simulink model "InjCrv_MI11"  (R2016b)
settings: configuration reference "CodeGenConfigSet" (kept outside this file)
values from neighbouring files (symbols this model uses):
  InjCrv_phiMI1Bas1EOM0_MAP = Calibration.Parameter    [init_InjCrv_MI1.m]    (also in init_InjCrv_MI1_SIL.m = Simulink.Parameter)
  InjCrv_phiMI1Bas1EOM0_MAPX = Calibration.Parameter    [init_InjCrv_MI1.m]    (also in init_InjCrv_MI1_SIL.m = Simulink.Parameter)
  InjCrv_phiMI1Bas1EOM0_MAPY = Calibration.Parameter    [init_InjCrv_MI1.m]    (also in init_InjCrv_MI1_SIL.m = Simulink.Parameter)
  InjCrv_phiMI1Bas2EOM0_MAP = Calibration.Parameter    [init_InjCrv_MI1.m]    (also in init_InjCrv_MI1_SIL.m = Simulink.Parameter)
  InjCrv_phiMI1Bas2EOM0_MAPX = Calibration.Parameter    [init_InjCrv_MI1.m]    (also in init_InjCrv_MI1_SIL.m = Simulink.Parameter)
  InjCrv_phiMI1Bas2EOM0_MAPY = Calibration.Parameter    [init_InjCrv_MI1.m]    (also in init_InjCrv_MI1_SIL.m = Simulink.Parameter)
  InjCrv_phiMI1Max1EOM0_MAP = Calibration.Parameter    [init_InjCrv_MI1.m]    (also in init_InjCrv_MI1_SIL.m = Simulink.Parameter)
  InjCrv_phiMI1Max1EOM0_MAPX = Calibration.Parameter    [init_InjCrv_MI1.m]    (also in init_InjCrv_MI1_SIL.m = Simulink.Parameter)
  InjCrv_phiMI1Max1EOM0_MAPY = Calibration.Parameter    [init_InjCrv_MI1.m]    (also in init_InjCrv_MI1_SIL.m = Simulink.Parameter)
  InjCrv_phiMI1Max2EOM0_MAP = Calibration.Parameter    [init_InjCrv_MI1.m]    (also in init_InjCrv_MI1_SIL.m = Simulink.Parameter)
  InjCrv_phiMI1Max2EOM0_MAPX = Calibration.Parameter    [init_InjCrv_MI1.m]    (also in init_InjCrv_MI1_SIL.m = Simulink.Parameter)
  InjCrv_phiMI1Max2EOM0_MAPY = Calibration.Parameter    [init_InjCrv_MI1.m]    (also in init_InjCrv_MI1_SIL.m = Simulink.Parameter)
  InjCrv_phiMI1Min_C = Calibration.Parameter    [init_InjCrv_MI1.m]    (also in init_InjCrv_MI1_SIL.m = Simulink.Parameter)
  InjCrv_phiMI1StrtBase_MAP = Calibration.Parameter    [init_InjCrv_MI1.m]    (also in init_InjCrv_MI1_SIL.m = Simulink.Parameter)
  InjCrv_phiMI1StrtBase_MAPX = Calibration.Parameter    [init_InjCrv_MI1.m]    (also in init_InjCrv_MI1_SIL.m = Simulink.Parameter)
  InjCrv_phiMI1StrtBase_MAPY = Calibration.Parameter    [init_InjCrv_MI1.m]    (also in init_InjCrv_MI1_SIL.m = Simulink.Parameter)
  InjCrv_qMI1Min_C = Calibration.Parameter    [init_InjCrv_MI1.m]    (also in init_InjCrv_MI1_SIL.m = Simulink.Parameter)
  InjCrv_qMI1MinPiIDiff_C = Calibration.Parameter    [init_InjCrv_MI1.m]    (also in init_InjCrv_MI1_SIL.m = Simulink.Parameter)
  InjCrv_qMI1MinPoIDiff_C = Calibration.Parameter    [init_InjCrv_MI1.m]    (also in init_InjCrv_MI1_SIL.m = Simulink.Parameter)
  InjCrv_stInjCharSetVal_C = Calibration.Parameter    [init_InjCrv_MI1.m]    (also in init_InjCrv_MI1_SIL.m = Simulink.Parameter)
  SigTst_phiMI1_C = Calibration.Parameter    [init_InjCrv_MI1.m]    (also in init_InjCrv_MI1_SIL.m = Simulink.Parameter)
  SigTst_qMI1_C = Calibration.Parameter    [init_InjCrv_MI1.m]    (also in init_InjCrv_MI1_SIL.m = Simulink.Parameter)
  SigTst_swtMI1Phi_C = Calibration.Parameter    [init_InjCrv_MI1.m]    (also in init_InjCrv_MI1_SIL.m = Simulink.Parameter)
  SigTst_swtMI1Q_C = Calibration.Parameter    [init_InjCrv_MI1.m]    (also in init_InjCrv_MI1_SIL.m = Simulink.Parameter)
undefined symbols (not defined in the file or in its folder): EngState_conv, Switch_conv
libraries: simulink x10, CXLib x3
settings Model: Creator=Administrator  LastModifiedBy=mayongchao
settings ConfigSetRef: SourceLocation=Base Workspace

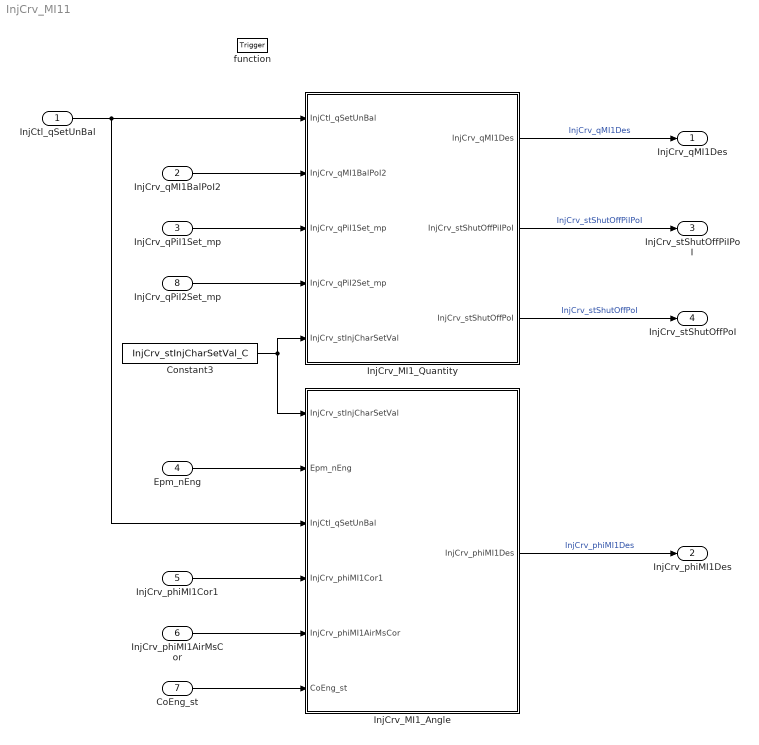
== system InjCrv_MI11 ==
  InjCtl_qSetUnBal : Inport  Tag=mg/hub  Description=Current injection quantity  OutMin=-319  OutMax=319  OutDataTypeStr=FuelMass_mg_hub
  InjCrv_qMI1BalPoI2 : Inport  Tag=mg/hub  Description=Actual PoI2 quantity contained in FMTC (used for MI1 balance)  Port=2  OutMin=-319  OutMax=319  OutDataTypeStr=FuelMass_mg_hub
  InjCrv_qPiI1Set_mp : Inport  Tag=mg/hub  Description=Set PiI1 quantity  Port=3  OutMin=-319  OutMax=319  OutDataTypeStr=FuelMass_mg_hub
  Epm_nEng : Inport  Tag=rpm  Description=Engine speed  Port=4  OutMin=0  OutMax=6000  OutDataTypeStr=EngSpeed_rpm
  InjCrv_phiMI1Cor1 : Inport  Tag=CA  Description=Start of energizing correction for MI1  Port=5  OutMin=-40  OutMax=40  OutDataTypeStr=Angle_CA
  InjCrv_phiMI1AirMsCor : Inport  Tag=CA  Description=The dynamic correction value is calculated as the compensation based on the air quality deviation  Port=6  OutMin=-10  OutMax=40  OutDataTypeStr=Angle_CA
  CoEng_st : Inport  Description=Engine coordinator state  Port=7  OutDataTypeStr=Enum: EngState_conv
  InjCrv_qPiI2Set_mp : Inport  Tag=mg/hub  Description=Set PiI2 quantity  Port=8  OutMin=-319  OutMax=319  OutDataTypeStr=FuelMass_mg_hub
  function : TriggerPort  TriggerType=function-call  VariantControl=Variant
  Constant3 : Constant  Value=InjCrv_stInjCharSetVal_C
  InjCrv_MI1_Angle : Subsystem
      settings: RTWSystemCode=Nonreusable function  RTWFileNameOpts=User specified
  InjCrv_MI1_Quantity : Subsystem
      settings: RTWSystemCode=Nonreusable function  RTWFileNameOpts=User specified
  InjCrv_qMI1Des : Outport  Tag=mg/hub  Description=desired MI1 injection quantity  OutMin=-319  OutMax=319  OutDataTypeStr=FuelMass_mg_hub
  InjCrv_phiMI1Des : Outport  Tag=CA  Description=Desired reference angle for the start of MI1  Port=2  OutMin=-40  OutMax=40  OutDataTypeStr=Angle_CA
  InjCrv_stShutOffPiIPoI : Outport  Description=State of MI1 fuelMass too small  Port=3  OutMin=0  OutMax=1  OutDataTypeStr=boolean
  InjCrv_stShutOffPoI : Outport  Description=State of MI1 fuelMass too small  Port=4  OutMin=0  OutMax=1  OutDataTypeStr=boolean
  wires:
  CoEng_st/1 -> InjCrv_MI1_Angle/6(CoEng_st)
  InjCrv_phiMI1AirMsCor/1 -> InjCrv_MI1_Angle/5(InjCrv_phiMI1AirMsCor)
  InjCrv_phiMI1Cor1/1 -> InjCrv_MI1_Angle/4(InjCrv_phiMI1Cor1)
  Epm_nEng/1 -> InjCrv_MI1_Angle/2(Epm_nEng)
  Constant3/1 -> InjCrv_MI1_Quantity/5(InjCrv_stInjCharSetVal), InjCrv_MI1_Angle/1(InjCrv_stInjCharSetVal)
  InjCtl_qSetUnBal/1 -> InjCrv_MI1_Angle/3(InjCtl_qSetUnBal), InjCrv_MI1_Quantity/1(InjCtl_qSetUnBal)
  InjCrv_qMI1BalPoI2/1 -> InjCrv_MI1_Quantity/2(InjCrv_qMI1BalPoI2)
  InjCrv_MI1_Quantity/1(InjCrv_qMI1Des) -> InjCrv_qMI1Des/1  "InjCrv_qMI1Des"
  InjCrv_MI1_Angle/1(InjCrv_phiMI1Des) -> InjCrv_phiMI1Des/1  "InjCrv_phiMI1Des"
  InjCrv_MI1_Quantity/2(InjCrv_stShutOffPiIPoI) -> InjCrv_stShutOffPiIPoI/1  "InjCrv_stShutOffPiIPoI"
  InjCrv_MI1_Quantity/3(InjCrv_stShutOffPoI) -> InjCrv_stShutOffPoI/1  "InjCrv_stShutOffPoI"
  InjCrv_qPiI1Set_mp/1 -> InjCrv_MI1_Quantity/3(InjCrv_qPiI1Set_mp)
  InjCrv_qPiI2Set_mp/1 -> InjCrv_MI1_Quantity/4(InjCrv_qPiI2Set_mp)

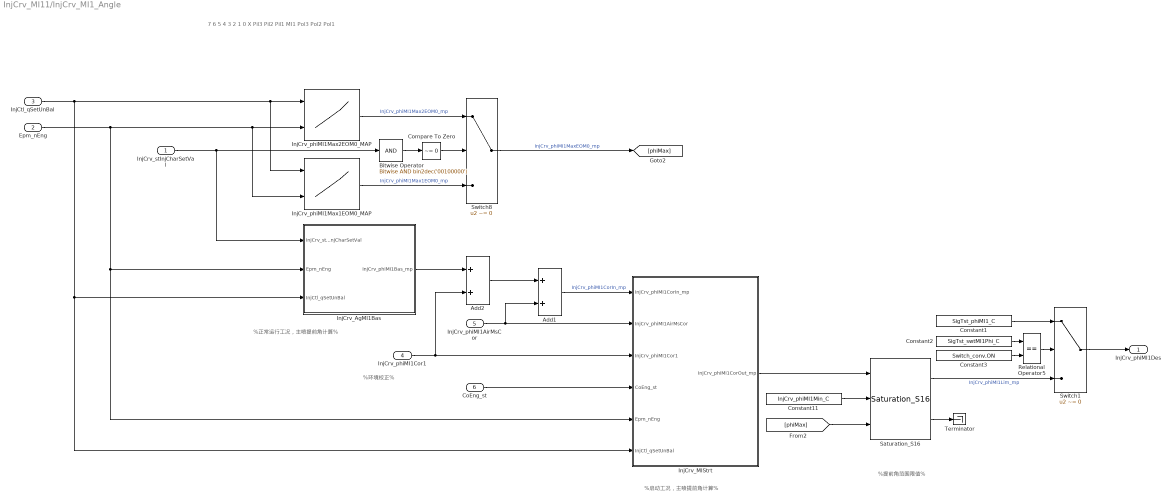
== system InjCrv_MI11/InjCrv_MI1_Angle ==
  note: 7
      | 6
      | 5
      | 4
      | 3
      | 2
      | 1
      | 0
      |
      | X
      | Pil3
      | Pil2
      | Pil1
      | MI1
      | Pol3
      | Pol2
      | Pol1
  note: %正常运行工况，主喷提前角计算%
  note: %启动工况，主喷提前角计算%
  note: %提前角范围限值%
  note: %环境校正%
  InjCrv_stInjCharSetVal : Inport
  Epm_nEng : Inport  Port=2
  InjCtl_qSetUnBal : Inport  Port=3
  InjCrv_phiMI1Cor1 : Inport  Port=4
  InjCrv_phiMI1AirMsCor : Inport  Port=5
  CoEng_st : Inport  Port=6
  Add1 : Sum  SaturateOnIntegerOverflow=on  InputSameDT=on
  Add2 : Sum  SaturateOnIntegerOverflow=on  InputSameDT=on
  Bitwise Operator : simulink/Logic and Bit Operations/Bitwise Operator  logicop=AND  UseBitMask=on  BitMask=bin2dec('00100000')  BitMaskRealWorld=Stored Integer
  Compare To Zero : simulink/Logic and Bit Operations/Compare To Zero  relop=~=  OutDataTypeStr=boolean
  Constant1 : Constant  Value=SigTst_phiMI1_C  SampleTime=-1
  Constant11 : Constant  Value=InjCrv_phiMI1Min_C
  Constant2 : Constant  Value=SigTst_swtMI1Phi_C
  Constant3 : Constant  RequirementInfo={'other' 'APP_requirements.doc' '@Simulink_requirement_item_25' 'true' '手动开关' '' } %GIDa_bc9d1e77_4373_4586_914d_b031e027f690  Value=Switch_conv.ON  OutDataTypeStr=Inherit: Inherit via back propagation
  InjCrv_AgMI1Bas : Subsystem
  InjCrv_MIStrt : Subsystem
  InjCrv_phiMI1Max1EOM0_MAP : Lookup_n-D  BreakpointsForDimension1=InjCrv_phiMI1Max1EOM0_MAPY  BreakpointsForDimension2=InjCrv_phiMI1Max1EOM0_MAPX  IndexSearchMethod=Linear search  BeginIndexSearchUsingPreviousIndexResult=on  Table=InjCrv_phiMI1Max1EOM0_MAP  ExtrapMethod=Clip  UseLastTableValue=on  InternalRulePriority=Speed  OutDataTypeStr=Inherit: Inherit via back propagation  SaturateOnIntegerOverflow=on
  InjCrv_phiMI1Max2EOM0_MAP : Lookup_n-D  BreakpointsForDimension1=InjCrv_phiMI1Max2EOM0_MAPY  BreakpointsForDimension2=InjCrv_phiMI1Max2EOM0_MAPX  IndexSearchMethod=Linear search  BeginIndexSearchUsingPreviousIndexResult=on  Table=InjCrv_phiMI1Max2EOM0_MAP  ExtrapMethod=Clip  UseLastTableValue=on  InternalRulePriority=Speed  OutDataTypeStr=Inherit: Inherit via back propagation  SaturateOnIntegerOverflow=on
  Relational Operator5 : RelationalOperator  Operator===  OutDataTypeStr=boolean  RndMeth=Simplest  InputSameDT=on
  Saturation_S16 : CXLib/Saturation_S16
  Switch1 : Switch  Criteria=u2 ~= 0  InputSameDT=on
  Switch8 : Switch  Criteria=u2 ~= 0  InputSameDT=on
  Terminator : Terminator
  InjCrv_phiMI1Des : Outport
  wires:
  Compare To Zero/1 -> Switch8/2
  Constant3/1 -> Relational Operator5/2
  Constant2/1 -> Relational Operator5/1
  Relational Operator5/1 -> Switch1/2
  Constant1/1 -> Switch1/1
  Constant11/1 -> Saturation_S16/2
  Bitwise Operator/1 -> Compare To Zero/1
  CoEng_st/1 -> InjCrv_MIStrt/4(CoEng_st)
  Switch1/1 -> InjCrv_phiMI1Des/1
  Saturation_S16/1 -> Switch1/3  "InjCrv_phiMI1Lim_mp"
  [phiMax] -> Saturation_S16/3
  InjCrv_MIStrt/1(InjCrv_phiMI1CorOut_mp) -> Saturation_S16/1
  Add1/1 -> InjCrv_MIStrt/1(InjCrv_phiMI1CorIn_mp)  "InjCrv_phiMI1CorIn_mp"
  Add2/1 -> Add1/1
  InjCrv_phiMI1AirMsCor/1 -> Add1/2, InjCrv_MIStrt/2(InjCrv_phiMI1AirMsCor)
  InjCrv_phiMI1Cor1/1 -> InjCrv_MIStrt/3(InjCrv_phiMI1Cor1), Add2/2
  InjCrv_AgMI1Bas/1(InjCrv_phiMI1Bas_mp) -> Add2/1
  Saturation_S16/2 -> Terminator/1
  Switch8/1 -> [phiMax]  "InjCrv_phiMI1MaxEOM0_mp"
  InjCtl_qSetUnBal/1 -> InjCrv_phiMI1Max1EOM0_MAP/1, InjCrv_phiMI1Max2EOM0_MAP/1, InjCrv_MIStrt/6(InjCtl_qSetUnBal), InjCrv_AgMI1Bas/3(InjCtl_qSetUnBal)
  Epm_nEng/1 -> InjCrv_phiMI1Max1EOM0_MAP/2, InjCrv_phiMI1Max2EOM0_MAP/2, InjCrv_MIStrt/5(Epm_nEng), InjCrv_AgMI1Bas/2(Epm_nEng)
  InjCrv_phiMI1Max2EOM0_MAP/1 -> Switch8/1  "InjCrv_phiMI1Max2EOM0_mp"
  InjCrv_phiMI1Max1EOM0_MAP/1 -> Switch8/3  "InjCrv_phiMI1Max1EOM0_mp"
  InjCrv_stInjCharSetVal/1 -> InjCrv_AgMI1Bas/1(InjCrv_stInjCharSetVal), Bitwise Operator/1

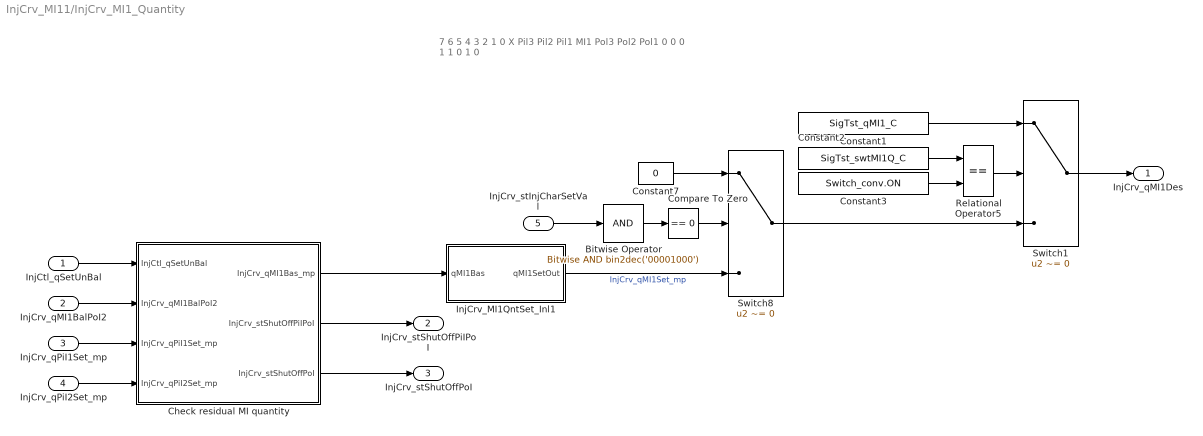
== system InjCrv_MI11/InjCrv_MI1_Quantity ==
  note: 7
      | 6
      | 5
      | 4
      | 3
      | 2
      | 1
      | 0
      |
      | X
      | Pil3
      | Pil2
      | Pil1
      | MI1
      | Pol3
      | Pol2
      | Pol1
      |
      | 0
      | 0
      | 0
      | 1
      | 1
      | 0
      | 1
      | 0
  InjCtl_qSetUnBal : Inport
  InjCrv_qMI1BalPoI2 : Inport  Port=2
  InjCrv_qPiI1Set_mp : Inport  Port=3
  InjCrv_qPiI2Set_mp : Inport  Port=4
  InjCrv_stInjCharSetVal : Inport  Port=5
  Bitwise Operator : simulink/Logic and Bit Operations/Bitwise Operator  logicop=AND  UseBitMask=on  BitMask=bin2dec('00001000')  BitMaskRealWorld=Stored Integer
  Check residual MI quantity : Subsystem
  Compare To Zero : simulink/Logic and Bit Operations/Compare To Zero  relop===  OutDataTypeStr=boolean
  Constant1 : Constant  Value=SigTst_qMI1_C
  Constant2 : Constant  Value=SigTst_swtMI1Q_C
  Constant3 : Constant  RequirementInfo={'other' 'APP_requirements.doc' '@Simulink_requirement_item_25' 'true' '手动开关' '' } %GIDa_5971a79d_3152_4918_9473_4b2de54e535e  Value=Switch_conv.ON  OutDataTypeStr=Inherit: Inherit via back propagation
  Constant7 : Constant  Value=0  OutDataTypeStr=Inherit: Inherit via back propagation
  InjCrv_MI1QntSet_Inl1 : Subsystem
  Relational Operator5 : RelationalOperator  Operator===  OutDataTypeStr=boolean  RndMeth=Round  InputSameDT=on
  Switch1 : Switch  Criteria=u2 ~= 0  OutDataTypeStr=Inherit: Inherit via back propagation  RndMeth=Round  InputSameDT=on
  Switch8 : Switch  Criteria=u2 ~= 0  OutDataTypeStr=Inherit: Inherit via back propagation  RndMeth=Round  InputSameDT=on
  InjCrv_qMI1Des : Outport
  InjCrv_stShutOffPiIPoI : Outport  Port=2
  InjCrv_stShutOffPoI : Outport  Port=3
  wires:
  Check residual MI quantity/3(InjCrv_stShutOffPoI) -> InjCrv_stShutOffPoI/1
  Check residual MI quantity/2(InjCrv_stShutOffPiIPoI) -> InjCrv_stShutOffPiIPoI/1
  InjCrv_qPiI1Set_mp/1 -> Check residual MI quantity/3(InjCrv_qPiI1Set_mp)
  InjCtl_qSetUnBal/1 -> Check residual MI quantity/1(InjCtl_qSetUnBal)
  InjCrv_qMI1BalPoI2/1 -> Check residual MI quantity/2(InjCrv_qMI1BalPoI2)
  Check residual MI quantity/1(InjCrv_qMI1Bas_mp) -> InjCrv_MI1QntSet_Inl1/1(qMI1Bas)
  Compare To Zero/1 -> Switch8/2
  Constant3/1 -> Relational Operator5/2
  Constant2/1 -> Relational Operator5/1
  Relational Operator5/1 -> Switch1/2
  Constant7/1 -> Switch8/1
  Constant1/1 -> Switch1/1
  Bitwise Operator/1 -> Compare To Zero/1
  Switch1/1 -> InjCrv_qMI1Des/1
  Switch8/1 -> Switch1/3
  InjCrv_stInjCharSetVal/1 -> Bitwise Operator/1
  InjCrv_MI1QntSet_Inl1/1(qMI1SetOut) -> Switch8/3  "InjCrv_qMI1Set_mp"
  InjCrv_qPiI2Set_mp/1 -> Check residual MI quantity/4(InjCrv_qPiI2Set_mp)

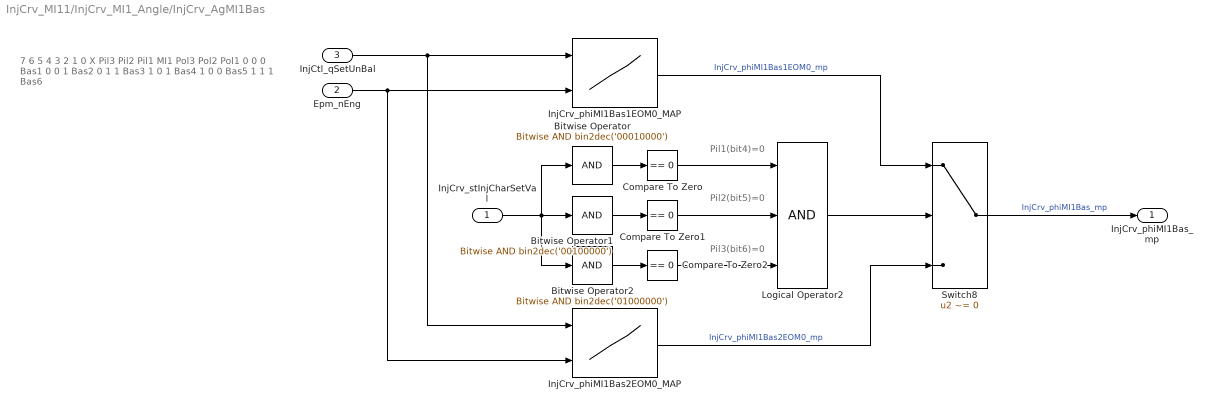
== system InjCrv_MI11/InjCrv_MI1_Angle/InjCrv_AgMI1Bas ==
  note: Pil1(bit4)=0
  note: Pil2(bit5)=0
  note: Pil3(bit6)=0
  note: 7
      | 6
      | 5
      | 4
      | 3
      | 2
      | 1
      | 0
      |
      | X
      | Pil3
      | Pil2
      | Pil1
      | MI1
      | Pol3
      | Pol2
      | Pol1
      |
      | 0
      | 0
      | 0
      | Bas1
      |
      | 0
      | 0
      | 1
      | Bas2
      |
      | 0
      | 1
      | 1
      | Bas3
      |
      | 1
      | 0
      | 1
      | Bas4
      |
      | 1
      | 0
      | 0
      | Bas5
      |
      | 1
      | 1
      | 1
      | Bas6
  InjCrv_stInjCharSetVal : Inport
  Epm_nEng : Inport  Port=2
  InjCtl_qSetUnBal : Inport  Port=3
  Bitwise Operator : simulink/Logic and Bit Operations/Bitwise Operator  logicop=AND  UseBitMask=on  BitMask=bin2dec('00010000')  BitMaskRealWorld=Stored Integer
  Bitwise Operator1 : simulink/Logic and Bit Operations/Bitwise Operator  logicop=AND  UseBitMask=on  BitMask=bin2dec('00100000')  BitMaskRealWorld=Stored Integer
  Bitwise Operator2 : simulink/Logic and Bit Operations/Bitwise Operator  logicop=AND  UseBitMask=on  BitMask=bin2dec('01000000')  BitMaskRealWorld=Stored Integer
  Compare To Zero : simulink/Logic and Bit Operations/Compare To Zero  relop===  OutDataTypeStr=boolean
  Compare To Zero1 : simulink/Logic and Bit Operations/Compare To Zero  relop===  OutDataTypeStr=boolean
  Compare To Zero2 : simulink/Logic and Bit Operations/Compare To Zero  relop===  OutDataTypeStr=boolean
  InjCrv_phiMI1Bas1EOM0_MAP : Lookup_n-D  BreakpointsForDimension1=InjCrv_phiMI1Bas1EOM0_MAPY  BreakpointsForDimension2=InjCrv_phiMI1Bas1EOM0_MAPX  IndexSearchMethod=Linear search  BeginIndexSearchUsingPreviousIndexResult=on  Table=InjCrv_phiMI1Bas1EOM0_MAP  ExtrapMethod=Clip  UseLastTableValue=on  InternalRulePriority=Speed  OutDataTypeStr=Inherit: Inherit via back propagation  SaturateOnIntegerOverflow=on
  InjCrv_phiMI1Bas2EOM0_MAP : Lookup_n-D  BreakpointsForDimension1=InjCrv_phiMI1Bas2EOM0_MAPY  BreakpointsForDimension2=InjCrv_phiMI1Bas2EOM0_MAPX  IndexSearchMethod=Linear search  BeginIndexSearchUsingPreviousIndexResult=on  Table=InjCrv_phiMI1Bas2EOM0_MAP  ExtrapMethod=Clip  UseLastTableValue=on  InternalRulePriority=Speed  OutDataTypeStr=Inherit: Inherit via back propagation  SaturateOnIntegerOverflow=on
  Logical Operator2 : Logic  Inputs=3  OutDataTypeStr=boolean
  Switch8 : Switch  Criteria=u2 ~= 0  InputSameDT=on
  InjCrv_phiMI1Bas_mp : Outport
  wires:
  Bitwise Operator2/1 -> Compare To Zero2/1
  Bitwise Operator1/1 -> Compare To Zero1/1
  Bitwise Operator/1 -> Compare To Zero/1
  Logical Operator2/1 -> Switch8/2
  Compare To Zero2/1 -> Logical Operator2/3
  Compare To Zero1/1 -> Logical Operator2/2
  Compare To Zero/1 -> Logical Operator2/1
  InjCrv_stInjCharSetVal/1 -> Bitwise Operator1/1, Bitwise Operator2/1, Bitwise Operator/1
  Switch8/1 -> InjCrv_phiMI1Bas_mp/1  "InjCrv_phiMI1Bas_mp"
  InjCtl_qSetUnBal/1 -> InjCrv_phiMI1Bas1EOM0_MAP/1, InjCrv_phiMI1Bas2EOM0_MAP/1
  Epm_nEng/1 -> InjCrv_phiMI1Bas1EOM0_MAP/2, InjCrv_phiMI1Bas2EOM0_MAP/2
  InjCrv_phiMI1Bas1EOM0_MAP/1 -> Switch8/1  "InjCrv_phiMI1Bas1EOM0_mp"
  InjCrv_phiMI1Bas2EOM0_MAP/1 -> Switch8/3  "InjCrv_phiMI1Bas2EOM0_mp"

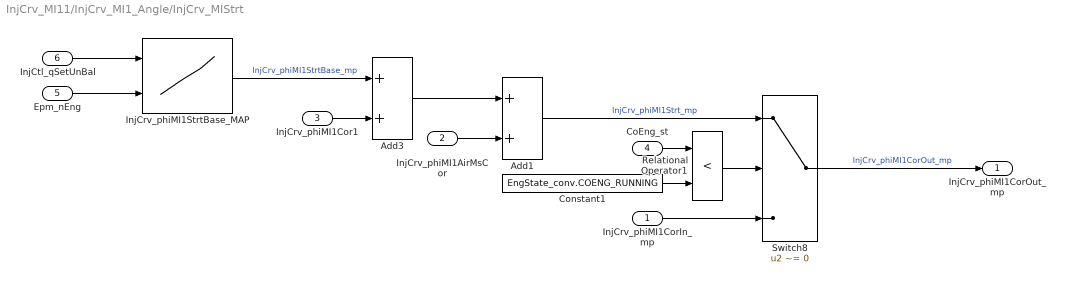
== system InjCrv_MI11/InjCrv_MI1_Angle/InjCrv_MIStrt ==
  InjCrv_phiMI1CorIn_mp : Inport
  InjCrv_phiMI1AirMsCor : Inport  Port=2
  InjCrv_phiMI1Cor1 : Inport  Port=3
  CoEng_st : Inport  Port=4
  Epm_nEng : Inport  Port=5
  InjCtl_qSetUnBal : Inport  Port=6
  Add1 : Sum  SaturateOnIntegerOverflow=on  InputSameDT=on
  Add3 : Sum  SaturateOnIntegerOverflow=on  InputSameDT=on
  Constant1 : Constant  Value=EngState_conv.COENG_RUNNING
  InjCrv_phiMI1StrtBase_MAP : Lookup_n-D  BreakpointsForDimension1=InjCrv_phiMI1StrtBase_MAPY  BreakpointsForDimension2=InjCrv_phiMI1StrtBase_MAPX  IndexSearchMethod=Linear search  BeginIndexSearchUsingPreviousIndexResult=on  Table=InjCrv_phiMI1StrtBase_MAP  ExtrapMethod=Clip  UseLastTableValue=on  InternalRulePriority=Speed  OutDataTypeStr=Inherit: Inherit via back propagation  SaturateOnIntegerOverflow=on
  Relational Operator1 : RelationalOperator  Operator=<  OutDataTypeStr=boolean  RndMeth=Nearest  InputSameDT=on
  Switch8 : Switch  Criteria=u2 ~= 0  InputSameDT=on
  InjCrv_phiMI1CorOut_mp : Outport
  wires:
  InjCtl_qSetUnBal/1 -> InjCrv_phiMI1StrtBase_MAP/1
  Epm_nEng/1 -> InjCrv_phiMI1StrtBase_MAP/2
  Add1/1 -> Switch8/1  "InjCrv_phiMI1Strt_mp"
  Add3/1 -> Add1/1
  InjCrv_phiMI1AirMsCor/1 -> Add1/2
  InjCrv_phiMI1CorIn_mp/1 -> Switch8/3
  Switch8/1 -> InjCrv_phiMI1CorOut_mp/1  "InjCrv_phiMI1CorOut_mp"
  CoEng_st/1 -> Relational Operator1/1
  Constant1/1 -> Relational Operator1/2
  Relational Operator1/1 -> Switch8/2
  InjCrv_phiMI1Cor1/1 -> Add3/2
  InjCrv_phiMI1StrtBase_MAP/1 -> Add3/1  "InjCrv_phiMI1StrtBase_mp"

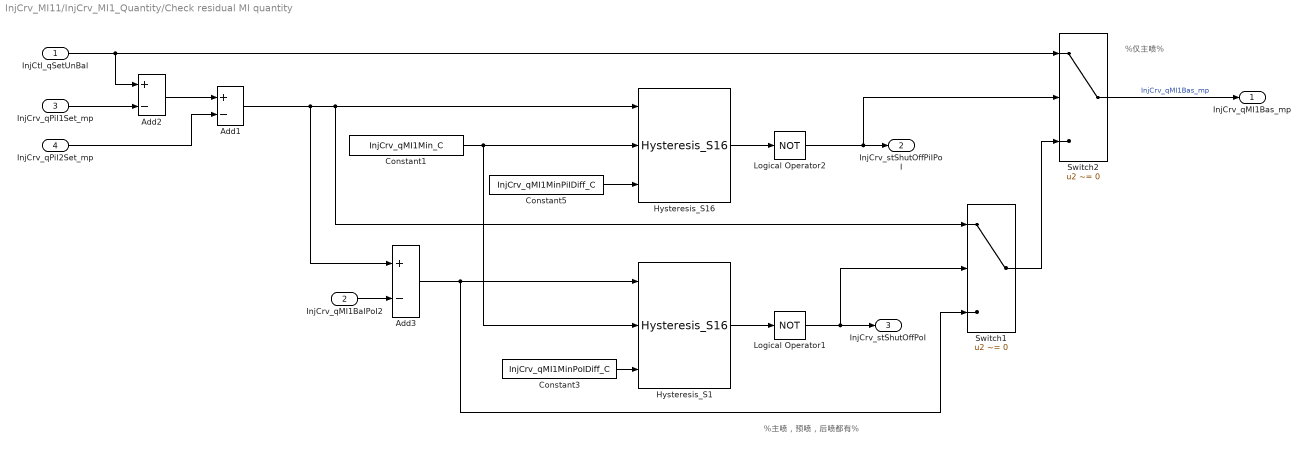
== system InjCrv_MI11/InjCrv_MI1_Quantity/Check residual MI quantity ==
  note: %仅主喷%
  note: %主喷，预喷，后喷都有%
  InjCtl_qSetUnBal : Inport
  InjCrv_qMI1BalPoI2 : Inport  Port=2
  InjCrv_qPiI1Set_mp : Inport  Port=3
  InjCrv_qPiI2Set_mp : Inport  Port=4
  Add1 : Sum  Inputs=+-  SaturateOnIntegerOverflow=on  InputSameDT=on
  Add2 : Sum  Inputs=+-  SaturateOnIntegerOverflow=on  InputSameDT=on
  Add3 : Sum  Inputs=+-  SaturateOnIntegerOverflow=on  InputSameDT=on
  Constant1 : Constant  Value=InjCrv_qMI1Min_C
  Constant3 : Constant  Value=InjCrv_qMI1MinPoIDiff_C
  Constant5 : Constant  Value=InjCrv_qMI1MinPiIDiff_C
  Hysteresis_S1 : CXLib/Hysteresis_S16
  Hysteresis_S16 : CXLib/Hysteresis_S16
  Logical Operator1 : Logic  Operator=NOT  Inputs=3  OutDataTypeStr=boolean
  Logical Operator2 : Logic  Operator=NOT  Inputs=3  OutDataTypeStr=boolean
  Switch1 : Switch  Criteria=u2 ~= 0  OutDataTypeStr=Inherit: Inherit via back propagation  RndMeth=Round  InputSameDT=on
  Switch2 : Switch  Criteria=u2 ~= 0  OutDataTypeStr=Inherit: Inherit via back propagation  RndMeth=Round  InputSameDT=on
  InjCrv_qMI1Bas_mp : Outport
  InjCrv_stShutOffPiIPoI : Outport  Port=2
  InjCrv_stShutOffPoI : Outport  Port=3
  wires:
  Add3/1 -> Switch1/3, Hysteresis_S1/1
  Logical Operator1/1 -> Switch1/2, InjCrv_stShutOffPoI/1
  Hysteresis_S1/1 -> Logical Operator1/1
  Switch1/1 -> Switch2/3
  Constant3/1 -> Hysteresis_S1/3
  Constant1/1 -> Hysteresis_S1/2, Hysteresis_S16/2
  Logical Operator2/1 -> Switch2/2, InjCrv_stShutOffPiIPoI/1
  Hysteresis_S16/1 -> Logical Operator2/1
  Add1/1 -> Add3/1, Switch1/1, Hysteresis_S16/1
  InjCrv_qMI1BalPoI2/1 -> Add3/2
  InjCrv_qPiI1Set_mp/1 -> Add2/2
  InjCtl_qSetUnBal/1 -> Switch2/1, Add2/1
  Constant5/1 -> Hysteresis_S16/3
  Switch2/1 -> InjCrv_qMI1Bas_mp/1  "InjCrv_qMI1Bas_mp"
  Add2/1 -> Add1/1
  InjCrv_qPiI2Set_mp/1 -> Add1/2

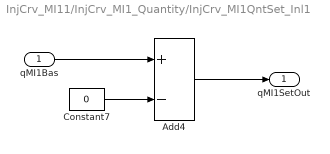
== system InjCrv_MI11/InjCrv_MI1_Quantity/InjCrv_MI1QntSet_Inl1 ==
  qMI1Bas : Inport
  Add4 : Sum  Inputs=+-  OutDataTypeStr=Inherit: Inherit via back propagation  SaturateOnIntegerOverflow=on  InputSameDT=on
  Constant7 : Constant  Value=0  OutDataTypeStr=Inherit: Inherit via back propagation
  qMI1SetOut : Outport
  wires:
  Constant7/1 -> Add4/2
  Add4/1 -> qMI1SetOut/1
  qMI1Bas/1 -> Add4/1
